simulink model "GPC_ss"  (R2020b)
settings: Solver=VariableStepAuto  StartTime=0.0  StopTime=14000  RelTol=1e-3
values from neighbouring files (symbols this model uses):
  b0 = 0.005    [madrc_2020_completo.m]
  beta1 = 3 * omega_o    (= 2.7)    [madrc_2020_completo.m]
  beta2 = 3 * omega_o^2    (= 2.43)    [madrc_2020_completo.m]
  beta3 = omega_o^3    (= 0.729)    [madrc_2020_completo.m]
  denominador_gcp = conv(den_poly_gcp, conv(den_poly_gcp, den_poly_gcp))    [madrc_2020_completo.m]
  denominador_real = conv(den_poly, conv(den_poly, conv(den_poly, conv(den_poly, den_poly))))    [madrc_2020_completo.m]
  kd = 2 * omega_c    (= 0.044)    [madrc_2020_completo.m]
  kp = omega_c^2    (= 0.000484)    [madrc_2020_completo.m]
  numerador_gcp = 1    [madrc_2020_completo.m]
  numerador_real = K    [madrc_2020_completo.m]
  ref_final = 26,4    [madrc_2020_completo.m]
  ref_inicial = 0    [madrc_2020_completo.m]
  t_degrau = 50    [madrc_2020_completo.m]
  Ts = 1    [madrc_2020_completo.m]
undefined symbols (not defined in the file or in its folder): A_ss, D, H, KE_ss, KF_ss, Kr_ss, Ts_ss
libraries: cstblocks x2
settings Model: Creator=LACER_GMG  LastModifiedBy=diego

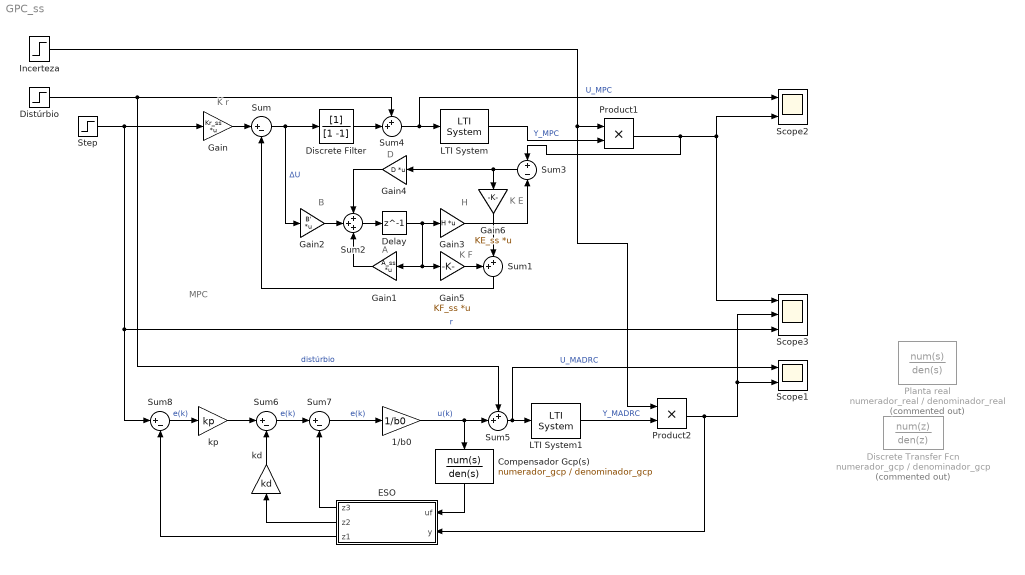
== system GPC_ss ==
  note: MPC
  note: D
  note: A
  note: B
  note: K F
  note: K E
  note: H
  note: K r
  1/b0 : Gain  Gain=1/b0
  Compensador Gcp(s) : TransferFcn  Numerator=numerador_gcp  Denominator=denominador_gcp
  Delay : Delay  DelayLength=1  InitialCondition=0  SampleTime=Ts_ss
  Discrete Transfer Fcn : DiscreteTransferFcn  Commented=on  Numerator=numerador_gcp  Denominator=denominador_gcp  SampleTime=Ts
  Discrete Filter : DiscreteFilter  Denominator=[1 -1]  FilterStructure=Direct form I  SampleTime=Ts_ss
  Distúrbio : Step  Time=5000  After=0.25  SampleTime=Ts_ss
  ESO : Subsystem
  Gain : Gain  Gain=Kr_ss  Multiplication=Matrix(K*u)
  Gain1 : Gain  Gain=A_ss  Multiplication=Matrix(K*u)
  Gain2 : Gain  Gain=B'  Multiplication=Matrix(K*u)
  Gain3 : Gain  Gain=H  Multiplication=Matrix(K*u)
  Gain4 : Gain  Gain=D  Multiplication=Matrix(K*u)
  Gain5 : Gain  Gain=KF_ss  Multiplication=Matrix(K*u)
  Gain6 : Gain  Gain=KE_ss  Multiplication=Matrix(K*u)
  Incerteza : Step  Time=8500  Before=1  After=1.1  SampleTime=Ts_ss
  LTI System : cstblocks/LTI System  sys=P  IC=[]
  LTI System1 : cstblocks/LTI System  sys=P  IC=[]
  Planta real : TransferFcn  Commented=on  Numerator=numerador_real  Denominator=denominador_real
  Product1 : Product
  Product2 : Product
  Scope1 : Scope  NumInputPorts=2
  Scope2 : Scope  NumInputPorts=2
  Scope3 : Scope  NumInputPorts=3
  Step : Step  Time=t_degrau  Before=ref_inicial  After=ref_final  SampleTime=Ts_ss
  Sum{,6..8} (4 alike) : Sum  Inputs=|+-
  Sum1 : Sum  Inputs=++|
  Sum2 : Sum  Inputs=+++
  Sum3 : Sum  Inputs=+|-
  Sum4 : Sum  Inputs=++|
  Sum5 : Sum  Inputs=++|
  kd : Gain  Gain=kd
  kp : Gain  Gain=kp
  wires:
  Discrete Filter/1 -> Sum4/2
  Sum1/1 -> Sum/2
  Gain2/1 -> Sum2/2
  Sum3/1 -> Gain6/1, Gain4/1
  Gain3/1 -> Sum3/2
  Delay/1 -> Gain3/1, Gain5/1, Gain1/1
  Gain4/1 -> Sum2/1
  Sum2/1 -> Delay/1
  Gain1/1 -> Sum2/3
  Gain5/1 -> Sum1/1
  Gain6/1 -> Sum1/2
  Gain/1 -> Sum/1
  Sum/1 -> Gain2/1, Discrete Filter/1  "ΔU"
  LTI System/1 -> Product1/2  "Y_MPC"
  Sum4/1 -> Scope2/1, LTI System/1  "U_MPC"
  Step/1 -> Gain/1, Sum8/1, Scope3/3  "r"
  1/b0/1 -> Compensador Gcp(s)/1, Sum5/2  "u(k)"
  Sum6/1 -> Sum7/1  "e(k)"
  kd/1 -> Sum6/2
  kp/1 -> Sum6/1
  Sum7/1 -> 1/b0/1  "e(k)"
  Sum5/1 -> LTI System1/1, Scope1/1  "U_MADRC"
  Distúrbio/1 -> Sum5/1, Sum4/1  "distúrbio"
  ESO/3(z1) -> Sum8/2
  Sum8/1 -> kp/1  "e(k)"
  ESO/2(z2) -> kd/1
  Compensador Gcp(s)/1 -> ESO/1(uf)
  ESO/1(z3) -> Sum7/2
  Product1/1 -> Sum3/1, Scope2/2, Scope3/1
  Incerteza/1 -> Product2/1, Product1/1
  Product2/1 -> ESO/2(y), Scope3/2, Scope1/2
  LTI System1/1 -> Product2/2  "Y_MADRC"

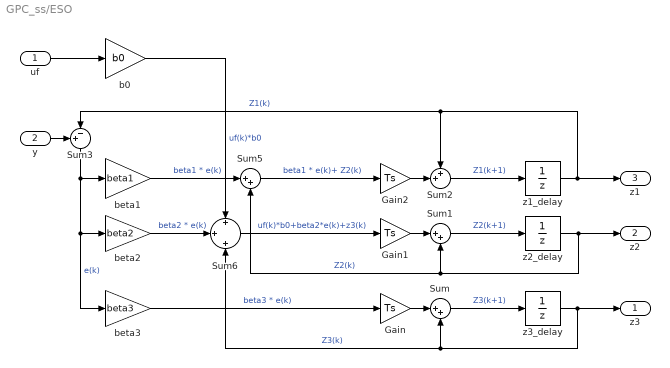
== system GPC_ss/ESO ==
  uf : Inport
  y : Inport  Port=2
  Gain : Gain  Gain=Ts
  Gain1 : Gain  Gain=Ts
  Gain2 : Gain  Gain=Ts
  Sum : Sum  Inputs=|++
  Sum1 : Sum  Inputs=|++
  Sum2 : Sum  Inputs=++|
  Sum3 : Sum  Inputs=+-|
  Sum5 : Sum  Inputs=|++
  Sum6 : Sum  Inputs=+|+|+
  b0 : Gain  Gain=b0
  beta1 : Gain  Gain=beta1
  beta2 : Gain  Gain=beta2
  beta3 : Gain  Gain=beta3
  z1_delay : UnitDelay  HasFrameUpgradeWarning=on
  z2_delay : UnitDelay  HasFrameUpgradeWarning=on
  z3_delay : UnitDelay  HasFrameUpgradeWarning=on
  z3 : Outport
  z2 : Outport  Port=2
  z1 : Outport  Port=3
  wires:
  Sum3/1 -> beta1/1, beta2/1, beta3/1  "e(k)"
  Sum6/1 -> Gain1/1  "uf(k)*b0+beta2*e(k)+z3(k)"
  beta2/1 -> Sum6/2  "beta2 * e(k)"
  z1_delay/1 -> z1/1, Sum3/2, Sum2/1  "Z1(k)"
  Gain1/1 -> Sum1/1
  Gain2/1 -> Sum2/2
  Sum2/1 -> z1_delay/1  "Z1(k+1)"
  beta3/1 -> Gain/1  "beta3 * e(k)"
  Sum5/1 -> Gain2/1  "beta1 * e(k)+ Z2(k)"
  beta1/1 -> Sum5/1  "beta1 * e(k)"
  Gain/1 -> Sum/1
  z3_delay/1 -> z3/1, Sum6/3, Sum/2  "Z3(k)"
  Sum1/1 -> z2_delay/1  "Z2(k+1)"
  z2_delay/1 -> z2/1, Sum5/2, Sum1/2  "Z2(k)"
  Sum/1 -> z3_delay/1  "Z3(k+1)"
  y/1 -> Sum3/1
  uf/1 -> b0/1
  b0/1 -> Sum6/1  "uf(k)*b0"
